simulink model "myRegenModel"  (R2024b)
settings: Solver=VariableStepAuto  StartTime=0.0  StopTime=10.0  RelTol=1e-3
libraries: mpclib x1, SignalEditorBlockLib x1
settings Model: Creator=nakht  LastModifiedBy=nakht

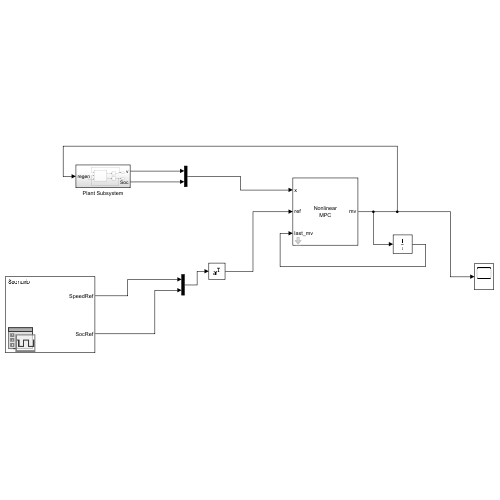
[thumbnail: Simulink's stored preview of the top-level diagram]
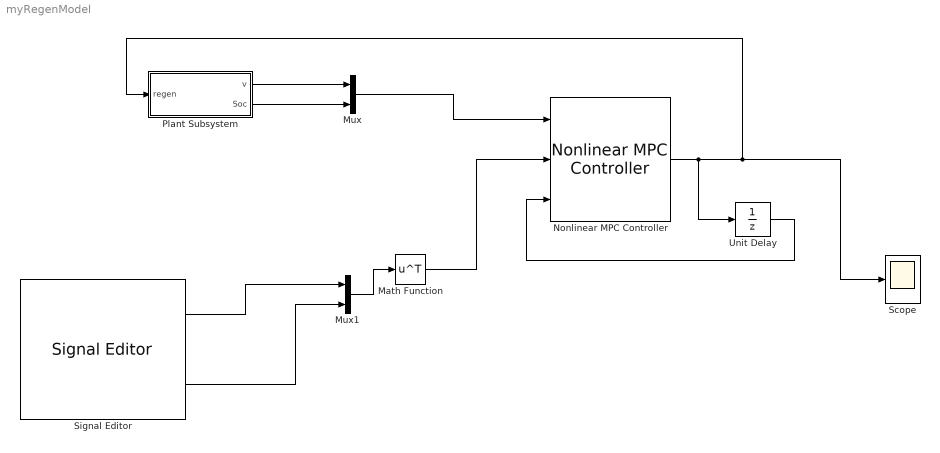
== system myRegenModel ==
  Math Function : Math  Operator=transpose
  Mux : Mux  Inputs=2
  Mux1 : Mux  Inputs=2
  Nonlinear MPC Controller : mpclib/Nonlinear MPC Controller  nlmpcobj=nlobj  UseObjectTs=off  TsControl=0.1  UseMEX=off  md_enabled=off  mvtarget_enabled=off  param_enabled=off  cost_enabled=off  mvseq_enabled=off  stateseq_enabled=off  ovseq_enabled=off  slack_enabled=off  status_enabled=off  ov_min=off  ov_max=off  mv_min=off  mv_max=off  mvrate_min=off  mvrate_max=off  state_min=off  state_max=off  ov_weight=off  mv_weight=off  mvrate_weight=off  ecr_weight=off  nlp_initialize=off
  Plant Subsystem : Subsystem
  Scope : Scope
  Signal Editor : SignalEditorBlockLib/Signal Editor  FileName=C:\Users\nakht\OneDrive\Documents\MATLAB\m1\ref.mat  ActiveScenario=Scenario  ActiveSignal=SpeedRef  IsBus=off  OutputBusObjectStr=Bus: BusObject  SampleTime=0  Interpolate=off  ZeroCross=off  OutputAfterFinalValue=Setting to zero  Unit=inherit  PreserveSignalName=on  ApplySigPropsToAllScenarios=on  ApplySigPropsToAllSignals=on
  Unit Delay : UnitDelay  SampleTime=-1  HasFrameUpgradeWarning=on
  wires:
  Nonlinear MPC Controller/1 -> Unit Delay/1, Scope/1, Plant Subsystem/1(regen)
  Plant Subsystem/1(v) -> Mux/1
  Plant Subsystem/2(Soc) -> Mux/2
  Mux/1 -> Nonlinear MPC Controller/1
  Unit Delay/1 -> Nonlinear MPC Controller/3
  Mux1/1 -> Math Function/1
  Math Function/1 -> Nonlinear MPC Controller/2
  Signal Editor/1 -> Mux1/1
  Signal Editor/2 -> Mux1/2

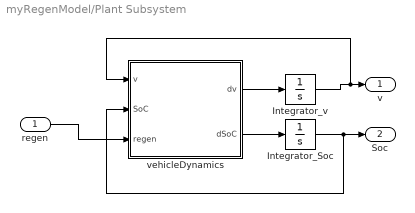
== system myRegenModel/Plant Subsystem ==
  regen : Inport
  Integrator_Soc : Integrator  InitialCondition=0.5
  Integrator_v : Integrator
  vehicleDynamics : MATLAB Function  TreatAsAtomicUnit=on
  v : Outport
  Soc : Outport  Port=2
  wires:
  vehicleDynamics/1(dv) -> Integrator_v/1
  Integrator_v/1 -> vehicleDynamics/1(v), v/1
  vehicleDynamics/2(dSoC) -> Integrator_Soc/1
  Integrator_Soc/1 -> vehicleDynamics/2(SoC), Soc/1
  regen/1 -> vehicleDynamics/3(regen)

== matlab function myRegenModel/Plant Subsystem/vehicleDynamics ==
  data: v input; dv output; SoC input; regen input; dSoC output
function [dv, dSoC] = vehicleDynamics(v, SoC, regen)
    % ODEs for the vehicle & battery:
    m       = 1000;
    r       = 0.3;
    rho     = 1.225;
    Cd      = 0.3;
    A       = 2.2;
    g       = 9.81;
    Crr     = 0.015;
    eta_chg = 0.8;
    Enom    = 1e5;

    dv   = -(1/m)*((regen/r) + 0.5*rho*Cd*A*v^2 + m*g*Crr);
    dSoC = eta_chg*(regen/Enom)*(v/r);
end
